simulink model "kde_old"  (R2022b)
settings: Solver=VariableStepAuto  StartTime=0.0  StopTime=orbit_E.T  FixedStep=1  RelTol=1e-9
values from neighbouring files (symbols this model uses):
  A0 = [1 0 0; 0 1 0; 0 0 1]    [test_script.m]
  gyro = struct('c', 15e-3, 'ARW', 0.15, 'sigma_b', deg2rad(0.3) / 3600,                'freq', 262, 'accuracy', 2.4e-9)    [test_script.m]
  H0 = sqrt((-29615e-9)^2+(-1728e-9)^2+(5186e-9)^2)    [test_script.m]
  I = [Ix; Iy; Iz]    [test_script.m]
  Ir = 0.005    [test_script.m]
  m_t = 5.9722e24    (= 5.9722e+24)    [test_script.m]
  Mr = 0    [test_script.m]
  orbit_E = struct('mu', astroConstants(13), 'a', astroConstants(23) + 2000,                    'e', 0.1, 'inc', deg2rad(10), 'G', astroConstants(1),                    'theta0', 0, 'R', astroConstants(23))    [test_script.m]
  orbit_S = struct('mu', astroConstants(4), 'a', astroConstants(2), 'e', 0.0167,                    'epsilon', deg2rad(23.45), 'G', astroConstants(1),                    'theta0', 0  )    [test_script.m]
  solarPanel = struct( 'r', r, 'P', radiation/(3e8),                      'rho_d', .1, 'rho_s', [.5, .5, .5, .5, .5 .5, .1, .1, .1, .1],                      'area', [.06 .06 .04 .06 .06 .04 .12 .12 .12 .12])    [test_script.m]
  w0 = [0; 0; orbit_E.n]    [test_script.m]
  wr0 = 0    [test_script.m]
undefined symbols (not defined in the file or in its folder): k1, k2
libraries: matrix_library x6, vrlib x2, dspinverses x1, simulink_extras x1
settings Model: Creator=stefa  LastModifiedBy=stefa
settings SolverCC: ZeroCrossAlgorithm=Adaptive

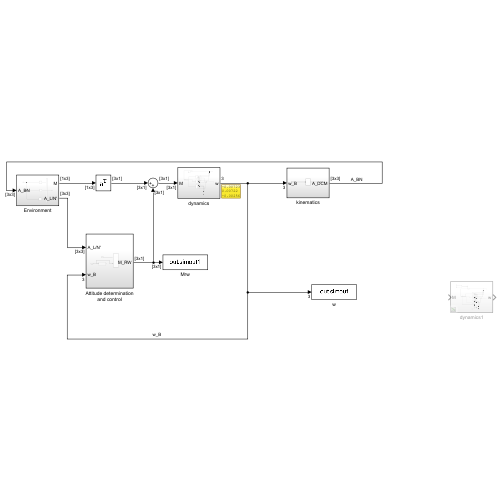
[thumbnail: Simulink's stored preview of the top-level diagram]
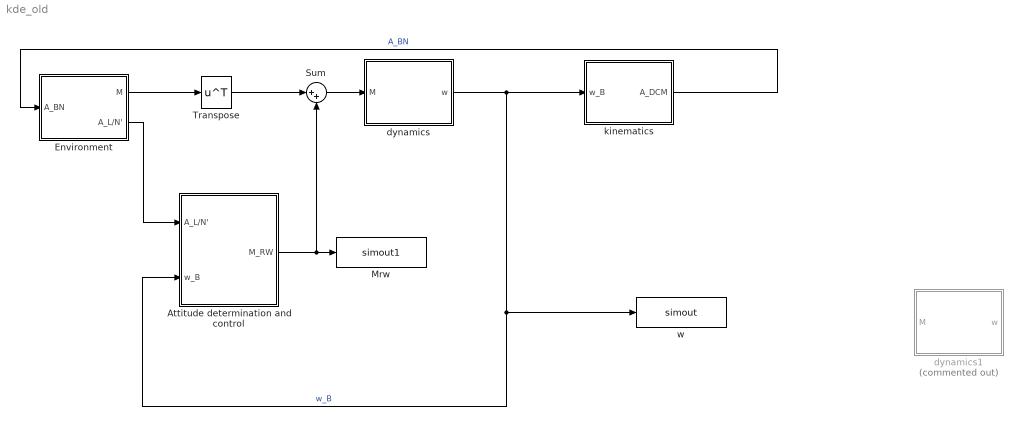
== system kde_old ==
  Attitude determination and control : Subsystem
  Environment : Subsystem
  Mrw : ToWorkspace  VariableName=simout1  SaveFormat=Timeseries  SampleTime=-1
  Sum : Sum  Inputs=|++
  Transpose : Math  Operator=transpose
  dynamics : Subsystem
  dynamics1 : Subsystem  Commented=on
  kinematics : Subsystem
  w : ToWorkspace  VariableName=simout  SaveFormat=Timeseries  SampleTime=-1
  wires:
  dynamics/1(w) -> kinematics/1(w_B), w/1, Attitude determination and control/2(w_B)  "w_B"
  kinematics/1(A_DCM) -> Environment/1(A_BN)  "A_BN"
  Sum/1 -> dynamics/1(M)
  Environment/2(A_L/N') -> Attitude determination and control/1(A_L/N')
  Attitude determination and control/1(M_RW) -> Mrw/1, Sum/2
  Environment/1(M) -> Transpose/1
  Transpose/1 -> Sum/1

== system kde_old/Attitude determination and control ==
  A_L/N' : Inport
  w_B : Inport  Port=2
  Actuator : Subsystem
  Sensors : Subsystem
  M_RW : Outport
  wires:
  A_L/N'/1 -> Actuator/1(A_L/N')
  Actuator/1(M_RW) -> M_RW/1
  w_B/1 -> Actuator/2(w_B), Sensors/1(w_B)
  Sensors/1(w_MB) -> Actuator/3(W_MB)

== system kde_old/Environment ==
  A_BN : Inport
  Magnetic field : Subsystem
  Sum : Sum  Inputs=+++
  gravity gradient : Subsystem
  srp disturbance : Subsystem
  M : Outport
  A_L/N' : Outport  Port=2
  wires:
  A_BN/1 -> Magnetic field/1(A_BN), srp disturbance/1(A_BN), gravity gradient/1(AB/N)
  Sum/1 -> M/1
  Magnetic field/1(M_B) -> Sum/1
  srp disturbance/1(M_srp) -> Sum/2
  gravity gradient/1(M_g) -> Sum/3
  gravity gradient/2(A_L/N') -> A_L/N'/1

== system kde_old/dynamics ==
  M : Inport
  Constant1 : Constant  Value=I
  Constant5 : Constant  Value=w0
  Demux : Demux  Outputs=3
  Demux1 : Demux  Outputs=3
  Demux2 : Demux  Outputs=3
  Integrator : Integrator  InitialConditionSource=external
  Mux : Mux  Inputs=3
  Subsystem : Subsystem
  Subsystem1 : Subsystem
  Subsystem2 : Subsystem
  w : Outport
  wires:
  Constant1/1 -> Demux1/1
  Demux1/2 -> Subsystem/4(Iy), Subsystem1/4(Iy), Subsystem2/4(Iy)  "Iy"
  Integrator/1 -> w/1, Demux/1  "w"
  Demux1/1 -> Subsystem/3(Ix), Subsystem1/3(Ix), Subsystem2/3(Ix)  "Ix"
  Demux2/2 -> Subsystem1/6(My)  "My"
  Demux1/3 -> Subsystem/5(Iz), Subsystem1/5(Iz), Subsystem2/5(Iz)  "Iz"
  Subsystem1/1(wy_dot) -> Mux/2
  Demux/1 -> Subsystem1/1(wx), Subsystem2/1(wx)  "wx"
  Subsystem2/1(wz_dot) -> Mux/3
  Demux2/3 -> Subsystem2/6(Mz)  "Mz"
  M/1 -> Demux2/1
  Demux/3 -> Subsystem1/2(wz), Subsystem/2(wz)  "wz"
  Demux/2 -> Subsystem2/2(wy), Subsystem/1(wy)  "wy"
  Demux2/1 -> Subsystem/6(Mx)  "Mx"
  Mux/1 -> Integrator/1  "w_dot"
  Subsystem/1(wx_dot) -> Mux/1
  Constant5/1 -> Integrator/2

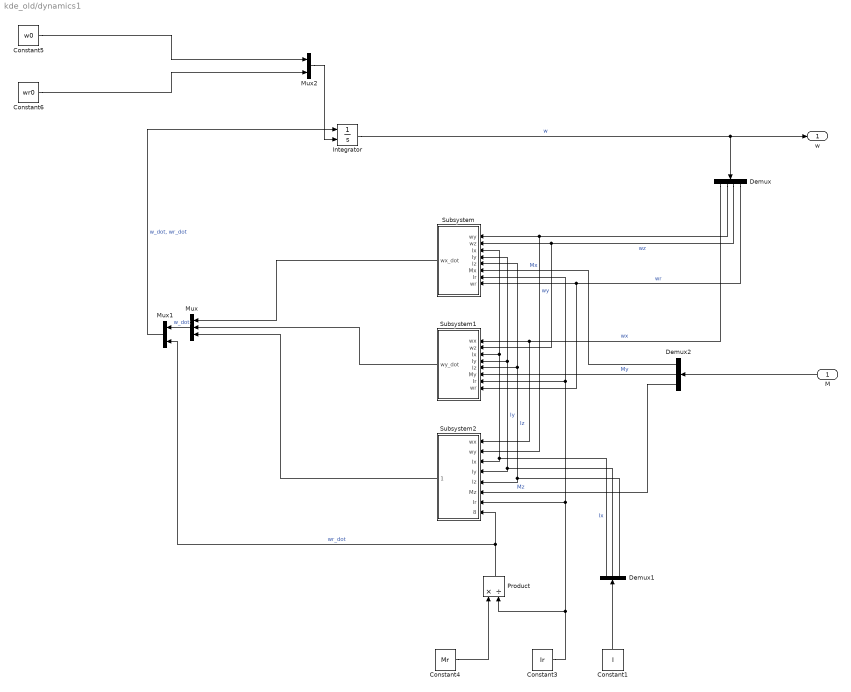
== system kde_old/dynamics1 ==
  M : Inport
  Constant1 : Constant  Value=I
  Constant3 : Constant  Value=Ir
  Constant4 : Constant  Value=Mr
  Constant5 : Constant  Value=w0
  Constant6 : Constant  Value=wr0
  Demux : Demux
  Demux1 : Demux  Outputs=3
  Demux2 : Demux  Outputs=3
  Integrator : Integrator  InitialConditionSource=external
  Mux : Mux  Inputs=3
  Mux1 : Mux  Inputs=2
  Mux2 : Mux  Inputs=2
  Product : Product  Inputs=*/
  Subsystem : Subsystem
  Subsystem1 : Subsystem
  Subsystem2 : Subsystem
  w : Outport
  wires:
  Constant1/1 -> Demux1/1
  Demux1/2 -> Subsystem/4(Iy), Subsystem1/4(Iy), Subsystem2/4(Iy)  "Iy"
  Integrator/1 -> w/1, Demux/1  "w"
  Demux1/1 -> Subsystem/3(Ix), Subsystem1/3(Ix), Subsystem2/3(Ix)  "Ix"
  Demux2/2 -> Subsystem1/6(My)  "My"
  Demux1/3 -> Subsystem/5(Iz), Subsystem1/5(Iz), Subsystem2/5(Iz)  "Iz"
  Subsystem1/1(wy_dot) -> Mux/2
  Demux/1 -> Subsystem1/1(wx), Subsystem2/1(wx)  "wx"
  Demux/4 -> Subsystem/8(wr), Subsystem1/8(wr)  "wr"
  Subsystem2/1(wz_dot) -> Mux/3
  Mux2/1 -> Integrator/2
  Demux2/3 -> Subsystem2/6(Mz)  "Mz"
  Constant6/1 -> Mux2/2
  M/1 -> Demux2/1
  Demux/3 -> Subsystem1/2(wz), Subsystem/2(wz)  "wz"
  Demux/2 -> Subsystem2/2(wy), Subsystem/1(wy)  "wy"
  Constant3/1 -> Product/2, Subsystem1/7(Ir), Subsystem/7(Ir), Subsystem2/7(Ir)
  Demux2/1 -> Subsystem/6(Mx)  "Mx"
  Mux1/1 -> Integrator/1  "w_dot, wr_dot"
  Product/1 -> Mux1/2, Subsystem2/8(wr_dot)  "wr_dot"
  Subsystem/1(wx_dot) -> Mux/1
  Constant5/1 -> Mux2/1
  Mux/1 -> Mux1/1  "w_dot"
  Constant4/1 -> Product/1

== system kde_old/kinematics ==
  w_B : Inport
  DCM : Subsystem
  A_DCM : Outport
  wires:
  w_B/1 -> DCM/1(w)
  DCM/1(A) -> A_DCM/1

== system kde_old/Attitude determination and control/Actuator ==
  A_L/N' : Inport
  w_B : Inport  Port=2
  W_MB : Inport  Port=3
  Constant : Constant  Value=[0 0 0]
  IdentityMatrix : IdentityMatrix  OutputDimensions=3
  IdentityMatrix1 : IdentityMatrix  OutputDimensions=3
  Reaction wheels : Subsystem
  Subsystem1 : Subsystem
  M_RW : Outport
  wires:
  IdentityMatrix/1 -> Reaction wheels/3(A)
  Reaction wheels/1(M_RW) -> M_RW/1
  Subsystem1/1(Mc) -> Reaction wheels/1(M_PD)
  Subsystem1/2(om) -> Reaction wheels/2(om)
  w_B/1 -> Subsystem1/2(w_MB)
  Constant/1 -> Subsystem1/3(w_target)
  IdentityMatrix1/1 -> Subsystem1/1(A_target)

== system kde_old/Attitude determination and control/Sensors ==
  w_B : Inport
  Constant : Constant  Commented=on  Value=gyro.c
  Constant1 : Constant  Commented=on  Value=gyro.A_eps
  MatrixMultiply1 : Product  Commented=on  Multiplication=Matrix(*)
  Product : Product  Commented=on
  noise : Subsystem
  w_MB : Outport
  wires:
  Product/1 -> MatrixMultiply1/1
  Constant1/1 -> Product/2
  Constant/1 -> Product/1
  noise/1(w_M) -> w_MB/1
  w_B/1 -> noise/1(C*A*w_B), MatrixMultiply1/2

== system kde_old/Environment/Magnetic field ==
  A_BN : Inport
  Cross Product : matrix_library/Cross Product
  Magnetic field : Subsystem
  m : Constant  Value=[0.01; 0.05; 0.01]
  M_B : Outport
  wires:
  A_BN/1 -> Magnetic field/1(A_BN)
  Magnetic field/1(b_B) -> Cross Product/2
  m/1 -> Cross Product/1
  Cross Product/1 -> M_B/1  "M_B"

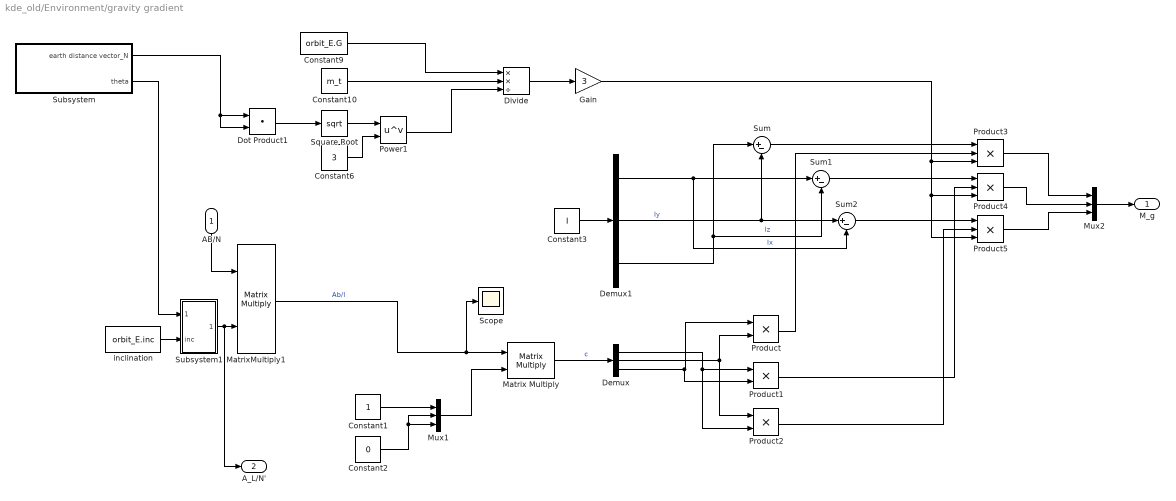
== system kde_old/Environment/gravity gradient ==
  AB/N : Inport
  Constant1 : Constant
  Constant10 : Constant  Value=m_t
  Constant2 : Constant  Value=0
  Constant3 : Constant  Value=I
  Constant6 : Constant  Value=3
  Constant9 : Constant  Value=orbit_E.G
  Demux : Demux  Outputs=3
  Demux1 : Demux  Outputs=3
  Divide : Product  Inputs=**/
  Dot Product1 : DotProduct  OutDataTypeStr=Inherit: Inherit via internal rule
  Gain : Gain  Gain=3
  Matrix Multiply : Product  Multiplication=Matrix(*)
  MatrixMultiply1 : Product  Multiplication=Matrix(*)
  Mux1 : Mux  Inputs=3
  Mux2 : Mux  Inputs=3
  Power1 : Math  Operator=pow
  Product : Product
  Product1 : Product
  Product2 : Product
  Product3 : Product  Inputs=3
  Product4 : Product  Inputs=3
  Product5 : Product  Inputs=3
  Scope : Scope
  Square Root : Sqrt
  Subsystem : Subsystem
  Subsystem1 : Subsystem
  Sum : Sum  Inputs=|+-
  Sum1 : Sum  Inputs=|+-
  Sum2 : Sum  Inputs=|+-
  inclination : Constant  Value=orbit_E.inc
  M_g : Outport
  A_L/N' : Outport  Port=2
  wires:
  AB/N/1 -> MatrixMultiply1/1
  MatrixMultiply1/1 -> Scope/1, Matrix Multiply/1  "Ab/l"
  Subsystem1/1(Al/n ') -> A_L/N'/1, MatrixMultiply1/2
  Subsystem/2(theta) -> Subsystem1/1(theta)
  Product4/1 -> Mux2/2
  Gain/1 -> Product5/3, Product4/3, Product3/3
  Demux1/2 -> Sum/2, Sum2/1  "Iy"
  Demux/3 -> Product1/2, Product/1
  Divide/1 -> Gain/1
  Demux1/3 -> Sum/1, Sum1/2  "Iz"
  Product1/1 -> Product4/2
  Constant1/1 -> Mux1/1
  Sum2/1 -> Product5/1
  Square Root/1 -> Power1/1
  Matrix Multiply/1 -> Demux/1  "c"
  Constant9/1 -> Divide/1
  Sum/1 -> Product3/1
  Demux/2 -> Product/2, Product2/1
  Constant6/1 -> Power1/2
  Product3/1 -> Mux2/1
  Mux1/1 -> Matrix Multiply/2
  Product/1 -> Product3/2
  Constant10/1 -> Divide/2
  Demux1/1 -> Sum2/2, Sum1/1  "Ix"
  Product2/1 -> Product5/2
  Constant2/1 -> Mux1/3, Mux1/2
  Product5/1 -> Mux2/3
  Demux/1 -> Product2/2, Product1/1
  Sum1/1 -> Product4/1
  Power1/1 -> Divide/3
  Dot Product1/1 -> Square Root/1
  Mux2/1 -> M_g/1
  Subsystem/1(earth distance vector_N) -> Dot Product1/2, Dot Product1/1
  Constant3/1 -> Demux1/1
  inclination/1 -> Subsystem1/2(inc)

== system kde_old/Environment/srp disturbance ==
  A_BN : Inport
  MatrixMultiply : Product  Multiplication=Matrix(*)
  Normalize Vector : vrlib/Utilities/Normalize Vector  maxzero=0
  Subsystem : Subsystem
  orientation s/c and solar panels : Subsystem
  sun distance magnitude : Subsystem
  M_srp : Outport
  wires:
  sun distance magnitude/1(S_N) -> Normalize Vector/1
  A_BN/1 -> MatrixMultiply/1
  Normalize Vector/1 -> MatrixMultiply/2
  Subsystem/1(M_SRP) -> M_srp/1
  orientation s/c and solar panels/1(N_B) -> Subsystem/2(N_B)
  MatrixMultiply/1 -> Subsystem/1(S_B)  "S_B"

== system kde_old/dynamics/Subsystem ==
  wy : Inport
  wz : Inport  Port=2
  Ix : Inport  Port=3
  Iy : Inport  Port=4
  Iz : Inport  Port=5
  Mx : Inport  Port=6
  Product : Product
  Product1 : Product
  Product3 : Product  Inputs=*/
  Sum : Sum  Inputs=|+-
  Sum1 : Sum  Inputs=|++
  wx_dot : Outport
  wires:
  Product1/1 -> Sum1/1
  Product/1 -> Product1/1
  Sum/1 -> Product1/2
  Product3/1 -> wx_dot/1  "wx_dot"
  Iy/1 -> Sum/1
  Iz/1 -> Sum/2
  wz/1 -> Product/1
  wy/1 -> Product/2
  Sum1/1 -> Product3/1
  Ix/1 -> Product3/2
  Mx/1 -> Sum1/2

== system kde_old/dynamics/Subsystem1 ==
  wx : Inport
  wz : Inport  Port=2
  Ix : Inport  Port=3
  Iy : Inport  Port=4
  Iz : Inport  Port=5
  My : Inport  Port=6
  Product : Product
  Product1 : Product
  Product3 : Product  Inputs=*/
  Sum : Sum  Inputs=|+-
  Sum2 : Sum  Inputs=|++
  wy_dot : Outport
  wires:
  Sum2/1 -> Product3/1
  Product1/1 -> Sum2/1
  Iy/1 -> Product3/2
  Sum/1 -> Product1/2
  Iz/1 -> Sum/1
  Product/1 -> Product1/1
  Product3/1 -> wy_dot/1
  Ix/1 -> Sum/2
  My/1 -> Sum2/2
  wz/1 -> Product/1
  wx/1 -> Product/2

== system kde_old/dynamics/Subsystem2 ==
  wx : Inport
  wy : Inport  Port=2
  Ix : Inport  Port=3
  Iy : Inport  Port=4
  Iz : Inport  Port=5
  Mz : Inport  Port=6
  Product : Product
  Product1 : Product
  Product3 : Product  Inputs=*/
  Sum : Sum  Inputs=|+-
  Sum1 : Sum  Inputs=|++
  wz_dot : Outport
  wires:
  Sum/1 -> Product1/2
  Product/1 -> Product1/1
  Iz/1 -> Product3/2
  Product3/1 -> wz_dot/1  "wz_dot"
  Sum1/1 -> Product3/1
  Product1/1 -> Sum1/1
  Ix/1 -> Sum/1
  wy/1 -> Product/1
  Iy/1 -> Sum/2
  Mz/1 -> Sum1/2
  wx/1 -> Product/2

== system kde_old/dynamics1/Subsystem ==
  wy : Inport
  wz : Inport  Port=2
  Ix : Inport  Port=3
  Iy : Inport  Port=4
  Iz : Inport  Port=5
  Mx : Inport  Port=6
  Ir : Inport  Port=7
  wr : Inport  Port=8
  Product : Product
  Product1 : Product
  Product2 : Product  Inputs=3
  Product3 : Product  Inputs=*/
  Sum : Sum  Inputs=|+-
  Sum1 : Sum  Inputs=|+-+
  wx_dot : Outport
  wires:
  Product1/1 -> Sum1/1
  Product/1 -> Product1/1
  Product2/1 -> Sum1/2
  Ir/1 -> Product2/2
  Sum/1 -> Product1/2
  Product3/1 -> wx_dot/1  "wx_dot"
  Iy/1 -> Sum/1
  Iz/1 -> Sum/2
  wz/1 -> Product/1
  Mx/1 -> Sum1/3
  wy/1 -> Product2/1, Product/2
  Sum1/1 -> Product3/1
  Ix/1 -> Product3/2
  wr/1 -> Product2/3

== system kde_old/dynamics1/Subsystem1 ==
  wx : Inport
  wz : Inport  Port=2
  Ix : Inport  Port=3
  Iy : Inport  Port=4
  Iz : Inport  Port=5
  My : Inport  Port=6
  Ir : Inport  Port=7
  wr : Inport  Port=8
  Product : Product
  Product1 : Product
  Product2 : Product  Inputs=3
  Product3 : Product  Inputs=*/
  Sum : Sum  Inputs=|+-
  Sum1 : Sum  Inputs=|++
  Sum2 : Sum  Inputs=|++
  wy_dot : Outport
  wires:
  Product1/1 -> Sum1/1
  Product2/1 -> Sum1/2
  Sum2/1 -> Product3/1
  Sum1/1 -> Sum2/1
  Iy/1 -> Product3/2
  Sum/1 -> Product1/2
  Iz/1 -> Sum/1
  Product/1 -> Product1/1
  Product3/1 -> wy_dot/1
  Ix/1 -> Sum/2
  My/1 -> Sum2/2
  wz/1 -> Product/1
  wx/1 -> Product2/1, Product/2
  wr/1 -> Product2/2
  Ir/1 -> Product2/3

== system kde_old/dynamics1/Subsystem2 ==
  wx : Inport
  wy : Inport  Port=2
  Ix : Inport  Port=3
  Iy : Inport  Port=4
  Iz : Inport  Port=5
  Mz : Inport  Port=6
  Ir : Inport  Port=7
  wr_dot : Inport  Port=8
  Product : Product
  Product1 : Product
  Product2 : Product
  Product3 : Product  Inputs=*/
  Sum : Sum  Inputs=|+-
  Sum1 : Sum  Inputs=|+-+
  wz_dot : Outport
  wires:
  Sum/1 -> Product1/2
  Product/1 -> Product1/1
  Iz/1 -> Product3/2
  Product3/1 -> wz_dot/1  "wz_dot"
  Sum1/1 -> Product3/1
  Product2/1 -> Sum1/2
  Product1/1 -> Sum1/1
  Ix/1 -> Sum/1
  wy/1 -> Product/1
  Iy/1 -> Sum/2
  Mz/1 -> Sum1/3
  Ir/1 -> Product2/1
  wx/1 -> Product/2
  wr_dot/1 -> Product2/2

== system kde_old/kinematics/DCM ==
  w : Inport
  Constant : Constant  Value=0
  Constant1 : Constant  Value=A0
  Gain : Gain  Gain=3/2
  Gain1 : Gain  Gain=1/2
  Integrator : Integrator  InitialConditionSource=external
  MatrixMultiply : Product  Multiplication=Matrix(*)
  MatrixMultiply1 : Product  Inputs=3  Multiplication=Matrix(*)
  Subsystem : Subsystem
  Sum : Sum  Inputs=|-+
  Transpose : Math  Operator=transpose
  A : Outport
  wires:
  Sum/1 -> A/1, MatrixMultiply/2
  Transpose/1 -> MatrixMultiply1/2
  MatrixMultiply/1 -> Integrator/1  "A_dot"
  Integrator/1 -> MatrixMultiply1/3, Gain/1, Transpose/1, MatrixMultiply1/1  "A"
  Subsystem/1(-[om^]) -> MatrixMultiply/1
  MatrixMultiply1/1 -> Gain1/1
  Constant/1 -> Subsystem/2(0)
  w/1 -> Subsystem/1(w)
  Constant1/1 -> Integrator/2
  Gain1/1 -> Sum/1
  Gain/1 -> Sum/2

== system kde_old/Attitude determination and control/Actuator/Reaction wheels ==
  M_PD : Inport
  om : Inport  Port=2
  A : Inport  Port=3
  Cross Product : matrix_library/Cross Product
  RW dynamics : Subsystem
  Sum : Sum  Inputs=|--
  M_RW : Outport
  wires:
  M_PD/1 -> RW dynamics/1(M_PD)
  om/1 -> Cross Product/1, RW dynamics/2(om)
  A/1 -> RW dynamics/3(A)
  RW dynamics/1(hr_dot) -> Sum/1
  RW dynamics/2(hr) -> Cross Product/2
  Cross Product/1 -> Sum/2
  Sum/1 -> M_RW/1

== system kde_old/Attitude determination and control/Actuator/Subsystem1 ==
  A_target : Inport
  w_MB : Inport  Port=2
  w_target : Inport  Port=3
  Constant : Constant  Value=I
  Constant1 : Constant  Value=k1
  Constant2 : Constant  Value=k2
  IdentityMatrix : IdentityMatrix  OutputDimensions=3
  Integrator : Integrator
  Integrator1 : Integrator  InitialConditionSource=external
  MATLAB Function : MATLAB Function  TreatAsAtomicUnit=on
  MATLAB Function1 : MATLAB Function  TreatAsAtomicUnit=on
  MATLAB Function2 : MATLAB Function  TreatAsAtomicUnit=on
  MatrixMultiply : Product  Multiplication=Matrix(*)
  Sum : Sum  Inputs=-+|
  Mc : Outport
  om : Outport  Port=2
  wires:
  Integrator/1 -> om/1, MATLAB Function1/1(om), MATLAB Function/3(om)
  MATLAB Function/1(om_dot) -> Integrator/1
  Constant/1 -> MATLAB Function/1(I)
  MATLAB Function1/1(dA) -> Integrator1/1
  Integrator1/1 -> MATLAB Function1/2(A), MatrixMultiply/1
  IdentityMatrix/1 -> Integrator1/2
  A_target/1 -> MatrixMultiply/2
  MatrixMultiply/1 -> MATLAB Function2/2(Ae)  "Ae"
  MATLAB Function2/1(u) -> MATLAB Function/2(u), Mc/1
  Constant1/1 -> MATLAB Function2/3(k1)
  Constant2/1 -> MATLAB Function2/4(k2)
  w_target/1 -> Sum/1
  w_MB/1 -> Sum/2
  Sum/1 -> MATLAB Function2/1(om)

== system kde_old/Attitude determination and control/Sensors/noise ==
  C*A*w_B : Inport
  Integrator : Integrator
  Sum : Sum  Inputs=+++
  b_dot : RandomNumber  Variance=(gyro.sigma_b) ^2  SampleTime=2000
  n : RandomNumber  Variance=(deg2rad(gyro.ARW)/60 * sqrt(gyro.freq))^2  SampleTime=2000
  w_M : Outport
  wires:
  b_dot/1 -> Integrator/1
  Sum/1 -> w_M/1
  n/1 -> Sum/2
  Integrator/1 -> Sum/3  "b"
  C*A*w_B/1 -> Sum/1

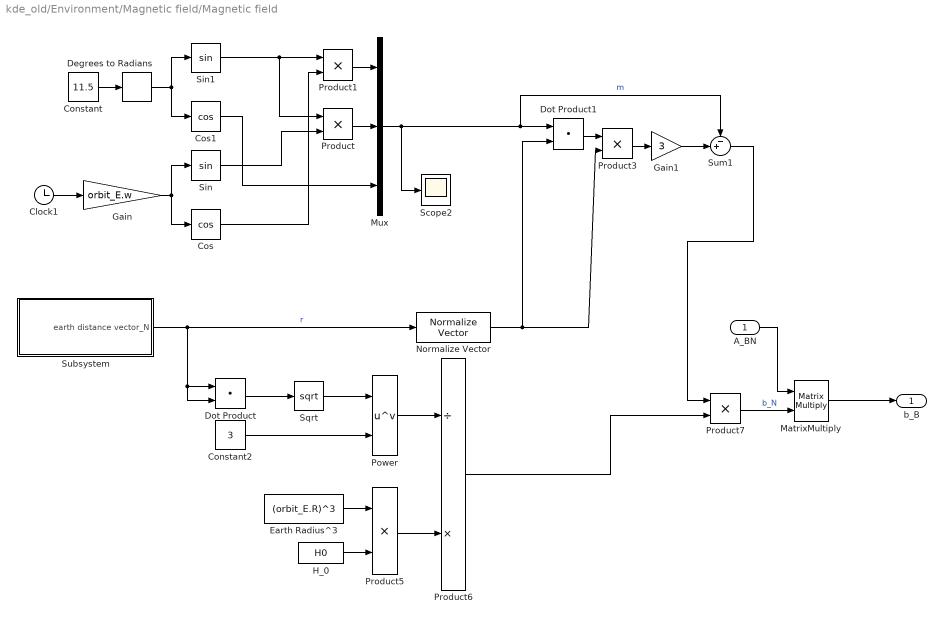
== system kde_old/Environment/Magnetic field/Magnetic field ==
  A_BN : Inport
  Clock1 : Clock
  Constant : Constant  Value=11.5
  Constant2 : Constant  Value=3
  Cos : Trigonometry  Operator=cos
  Cos1 : Trigonometry  Operator=cos
  Degrees to Radians : simulink_extras/Transformations/Degrees to Radians
  Dot Product : DotProduct  OutDataTypeStr=Inherit: Inherit via internal rule
  Dot Product1 : DotProduct  OutDataTypeStr=Inherit: Inherit via internal rule
  Earth Radius^3 : Constant  Value=(orbit_E.R)^3
  Gain : Gain  Gain=orbit_E.w
  Gain1 : Gain  Gain=3
  H_0 : Constant  Value=H0
  MatrixMultiply : Product  Multiplication=Matrix(*)
  Mux : Mux  Inputs=3
  Normalize Vector : vrlib/Utilities/Normalize Vector  maxzero=0
  Power : Math  Operator=pow
  Product{,1,3,5,7} (5 alike) : Product
  Product6 : Product  Inputs=/*
  Scope2 : Scope
  Sin : Trigonometry
  Sin1 : Trigonometry
  Sqrt : Sqrt
  Subsystem : Subsystem
  Sum1 : Sum  Inputs=-+|
  b_B : Outport
  wires:
  Constant2/1 -> Power/2
  Clock1/1 -> Gain/1
  Product1/1 -> Mux/1
  H_0/1 -> Product5/2
  Gain/1 -> Cos/1, Sin/1
  Subsystem/1(earth distance vector_N) -> Normalize Vector/1, Dot Product/1, Dot Product/2  "r"
  Mux/1 -> Dot Product1/1, Sum1/1, Scope2/1  "m"
  Dot Product/1 -> Sqrt/1
  Power/1 -> Product6/1
  Normalize Vector/1 -> Dot Product1/2, Product3/2
  Product6/1 -> Product7/2
  Dot Product1/1 -> Product3/1
  Product3/1 -> Gain1/1
  Degrees to Radians/1 -> Cos1/1, Sin1/1
  Cos1/1 -> Mux/3
  Product5/1 -> Product6/2
  Earth Radius^3/1 -> Product5/1
  Product/1 -> Mux/2
  Constant/1 -> Degrees to Radians/1
  Sin1/1 -> Product/1, Product1/1
  Sin/1 -> Product/2
  Product7/1 -> MatrixMultiply/2  "b_N"
  A_BN/1 -> MatrixMultiply/1
  MatrixMultiply/1 -> b_B/1
  Sqrt/1 -> Power/1
  Cos/1 -> Product1/2
  Sum1/1 -> Product7/1
  Gain1/1 -> Sum1/2

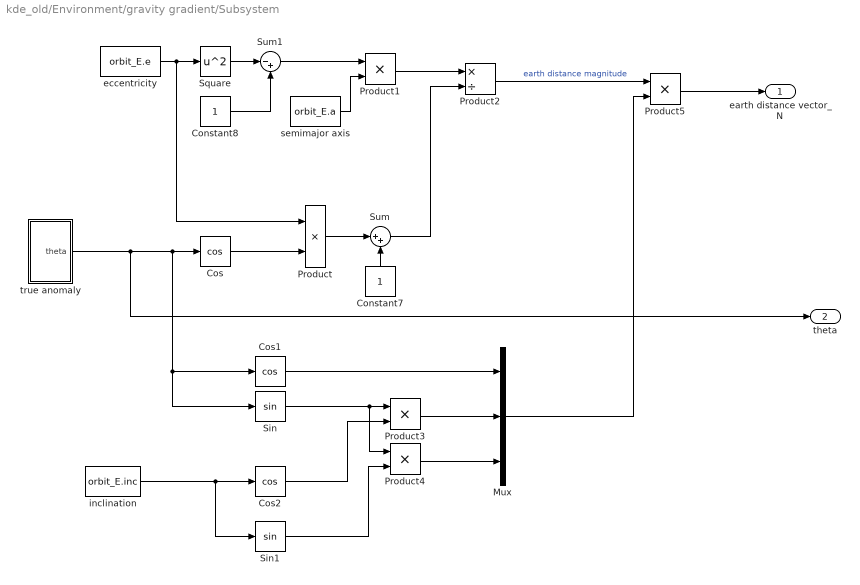
== system kde_old/Environment/gravity gradient/Subsystem ==
  Constant7 : Constant
  Constant8 : Constant
  Cos : Trigonometry  Operator=cos
  Cos1 : Trigonometry  Operator=cos
  Cos2 : Trigonometry  Operator=cos
  Mux : Mux  Inputs=3
  Product{,1,3..5} (5 alike) : Product
  Product2 : Product  Inputs=*/
  Sin : Trigonometry
  Sin1 : Trigonometry
  Square : Math  Operator=square
  Sum : Sum  Inputs=|++
  Sum1 : Sum  Inputs=|-+
  eccentricity : Constant  Value=orbit_E.e
  inclination : Constant  Value=orbit_E.inc
  semimajor axis : Constant  Value=orbit_E.a
  true anomaly : Subsystem
  earth distance vector_N : Outport
  theta : Outport  Port=2
  wires:
  Mux/1 -> Product5/2
  Product2/1 -> Product5/1  "earth distance magnitude"
  Product1/1 -> Product2/1
  Constant8/1 -> Sum1/2
  Sin/1 -> Product3/1, Product4/1
  true anomaly/1(theta) -> theta/1, Sin/1, Cos1/1, Cos/1
  Cos/1 -> Product/2
  eccentricity/1 -> Product/1, Square/1
  Sin1/1 -> Product4/2
  Sum1/1 -> Product1/1
  Sum/1 -> Product2/2
  Product3/1 -> Mux/2
  Cos1/1 -> Mux/1
  Square/1 -> Sum1/1
  semimajor axis/1 -> Product1/2
  inclination/1 -> Sin1/1, Cos2/1
  Product4/1 -> Mux/3
  Constant7/1 -> Sum/2
  Product/1 -> Sum/1
  Product5/1 -> earth distance vector_N/1
  Cos2/1 -> Product3/2

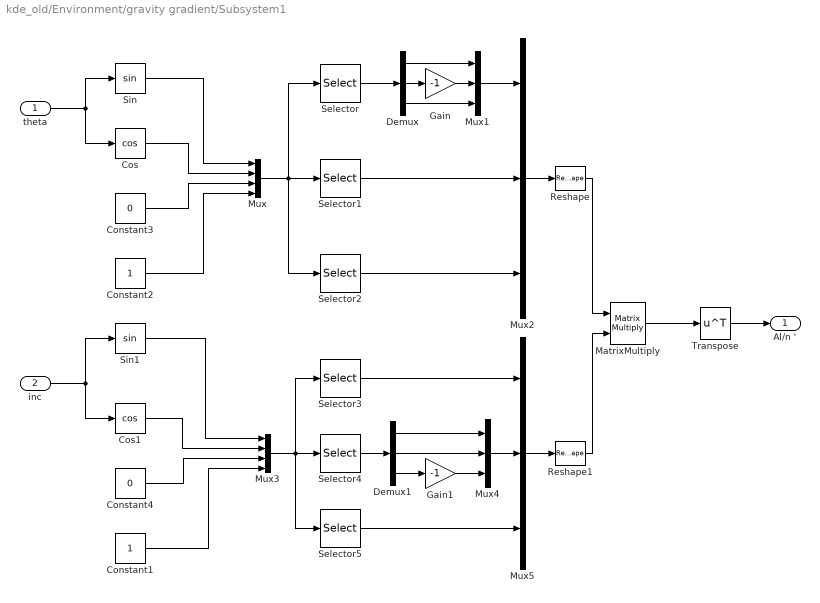
== system kde_old/Environment/gravity gradient/Subsystem1 ==
  theta : Inport
  inc : Inport  Port=2
  Constant1 : Constant
  Constant2 : Constant
  Constant3 : Constant  Value=0
  Constant4 : Constant  Value=0
  Cos : Trigonometry  Operator=cos
  Cos1 : Trigonometry  Operator=cos
  Demux : Demux  Outputs=3
  Demux1 : Demux  Outputs=3
  Gain : Gain  Gain=-1
  Gain1 : Gain  Gain=-1
  MatrixMultiply : Product  Multiplication=Matrix(*)
  Mux : Mux
  Mux{1..2,4..5} (4 alike) : Mux  Inputs=3
  Mux3 : Mux
  Reshape : Reshape  OutputDimensionality=Customize  OutputDimensions=[3,3]
  Reshape1 : Reshape  OutputDimensionality=Customize  OutputDimensions=[3,3]
  Selector : Selector  InputPortWidth=4  IndexOptions=Index vector (dialog)  Indices=[2 1 3]  OutputSizes=1
  Selector1 : Selector  InputPortWidth=4  IndexOptions=Index vector (dialog)  Indices=[1 2 3]  OutputSizes=1
  Selector2 : Selector  InputPortWidth=4  IndexOptions=Index vector (dialog)  Indices=[3 3 4]  OutputSizes=1
  Selector3 : Selector  InputPortWidth=4  IndexOptions=Index vector (dialog)  Indices=[4 3 3]  OutputSizes=1
  Selector4 : Selector  InputPortWidth=4  IndexOptions=Index vector (dialog)  Indices=[3 2 1]  OutputSizes=1
  Selector5 : Selector  InputPortWidth=4  IndexOptions=Index vector (dialog)  Indices=[3 1 2]  OutputSizes=1
  Sin : Trigonometry
  Sin1 : Trigonometry
  Transpose : Math  Operator=transpose
  Al/n ' : Outport
  wires:
  Constant2/1 -> Mux/4
  Constant3/1 -> Mux/3
  theta/1 -> Cos/1, Sin/1
  Cos/1 -> Mux/2
  Sin/1 -> Mux/1
  Mux/1 -> Selector2/1, Selector1/1, Selector/1
  Selector/1 -> Demux/1
  Demux/2 -> Gain/1
  Gain/1 -> Mux1/2
  Demux/3 -> Mux1/3
  Demux/1 -> Mux1/1
  Selector2/1 -> Mux2/3
  Mux1/1 -> Mux2/1
  Selector1/1 -> Mux2/2
  Mux2/1 -> Reshape/1
  Cos1/1 -> Mux3/2
  Sin1/1 -> Mux3/1
  Constant4/1 -> Mux3/3
  Constant1/1 -> Mux3/4
  inc/1 -> Cos1/1, Sin1/1
  Selector4/1 -> Demux1/1
  Demux1/3 -> Gain1/1
  Demux1/2 -> Mux4/2
  Demux1/1 -> Mux4/1
  Gain1/1 -> Mux4/3
  Mux3/1 -> Selector3/1, Selector4/1, Selector5/1
  Mux4/1 -> Mux5/2
  Selector3/1 -> Mux5/1
  Selector5/1 -> Mux5/3
  Mux5/1 -> Reshape1/1
  Reshape/1 -> MatrixMultiply/1
  Reshape1/1 -> MatrixMultiply/2
  MatrixMultiply/1 -> Transpose/1
  Transpose/1 -> Al/n '/1

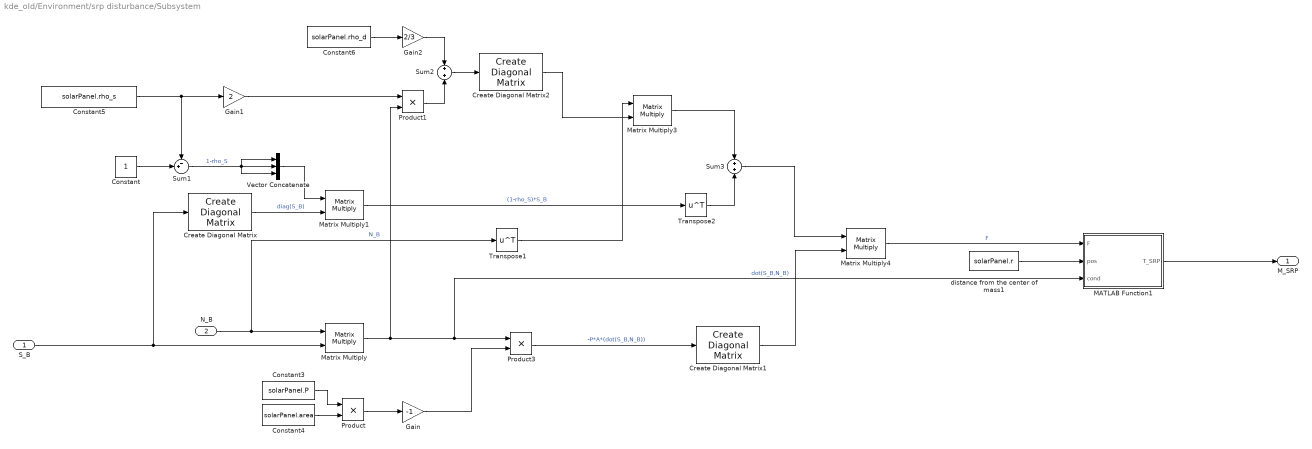
== system kde_old/Environment/srp disturbance/Subsystem ==
  S_B : Inport
  N_B : Inport  Port=2
  Constant : Constant
  Constant3 : Constant  Value=solarPanel.P
  Constant4 : Constant  Value=solarPanel.area
  Constant5 : Constant  Value=solarPanel.rho_s
  Constant6 : Constant  Value=solarPanel.rho_d
  Create Diagonal Matrix : matrix_library/Create Diagonal Matrix
      settings: LibrarySourceBlock=|
      | simulink/Matrix
      | Operations/Create Diagonal
      | Matrix
  Create Diagonal Matrix1 : matrix_library/Create Diagonal Matrix
      settings: LibrarySourceBlock=|
      | simulink/Matrix
      | Operations/Create Diagonal
      | Matrix
  Create Diagonal Matrix2 : matrix_library/Create Diagonal Matrix
      settings: LibrarySourceBlock=|
      | simulink/Matrix
      | Operations/Create Diagonal
      | Matrix
  Gain : Gain  Gain=-1
  Gain1 : Gain  Gain=2
  Gain2 : Gain  Gain=2/3
  MATLAB Function1 : MATLAB Function  TreatAsAtomicUnit=on
  Matrix Multiply{,1,3..4} (4 alike) : Product  Multiplication=Matrix(*)
  Product : Product
  Product1 : Product
  Product3 : Product
  Sum1 : Sum  Inputs=-+|
  Sum2 : Sum
  Sum3 : Sum
  Transpose1 : Math  Operator=transpose
  Transpose2 : Math  Operator=transpose
  Vector Concatenate : Concatenate  NumInputs=3  Mode=Multidimensional array  ConcatenateDimension=2
  distance from the center of mass1 : Constant  Value=solarPanel.r
  M_SRP : Outport
  wires:
  MATLAB Function1/1(T_SRP) -> M_SRP/1
  Create Diagonal Matrix1/1 -> Matrix Multiply4/2
  Product/1 -> Gain/1
  Matrix Multiply3/1 -> Sum3/1
  Product1/1 -> Sum2/2
  Transpose2/1 -> Sum3/2
  S_B/1 -> Create Diagonal Matrix/1, Matrix Multiply/2
  Constant4/1 -> Product/2
  Create Diagonal Matrix2/1 -> Matrix Multiply3/2
  Gain2/1 -> Sum2/1
  Constant/1 -> Sum1/2
  Matrix Multiply4/1 -> MATLAB Function1/1(F)  "F"
  Sum2/1 -> Create Diagonal Matrix2/1
  Product3/1 -> Create Diagonal Matrix1/1  "-P*A*(dot(S_B,N_B))"
  Create Diagonal Matrix/1 -> Matrix Multiply1/2  "diag(S_B)"
  N_B/1 -> Transpose1/1, Matrix Multiply/1  "N_B"
  Constant3/1 -> Product/1
  distance from the center of mass1/1 -> MATLAB Function1/2(pos)
  Matrix Multiply1/1 -> Transpose2/1  "(1-rho_S)*S_B"
  Constant5/1 -> Gain1/1, Sum1/1
  Gain/1 -> Product3/2
  Constant6/1 -> Gain2/1
  Sum1/1 -> Vector Concatenate/1, Vector Concatenate/3, Vector Concatenate/2  "1-rho_S"
  Gain1/1 -> Product1/1
  Sum3/1 -> Matrix Multiply4/1
  Matrix Multiply/1 -> Product1/2, MATLAB Function1/3(cond), Product3/1  "dot(S_B,N_B)"
  Vector Concatenate/1 -> Matrix Multiply1/1
  Transpose1/1 -> Matrix Multiply3/1

== system kde_old/Environment/srp disturbance/orientation s//c and solar panels ==
  Transpose : Math  Operator=transpose
  Vector Concatenate : Concatenate  NumInputs=10  Mode=Multidimensional array  ConcatenateDimension=2
  orientation s/c and solar panels in B : Subsystem
  N_B : Outport
  wires:
  orientation s/c and solar panels in B/6(n6) -> Vector Concatenate/6
  orientation s/c and solar panels in B/7(n7) -> Vector Concatenate/7
  orientation s/c and solar panels in B/3(n3) -> Vector Concatenate/3
  orientation s/c and solar panels in B/5(n5) -> Vector Concatenate/5
  orientation s/c and solar panels in B/10(n10) -> Vector Concatenate/10
  orientation s/c and solar panels in B/2(n2) -> Vector Concatenate/2
  orientation s/c and solar panels in B/8(n8) -> Vector Concatenate/8
  orientation s/c and solar panels in B/1(n1) -> Vector Concatenate/1
  orientation s/c and solar panels in B/4(n4) -> Vector Concatenate/4
  orientation s/c and solar panels in B/9(n9) -> Vector Concatenate/9
  Vector Concatenate/1 -> Transpose/1  "N_B"
  Transpose/1 -> N_B/1

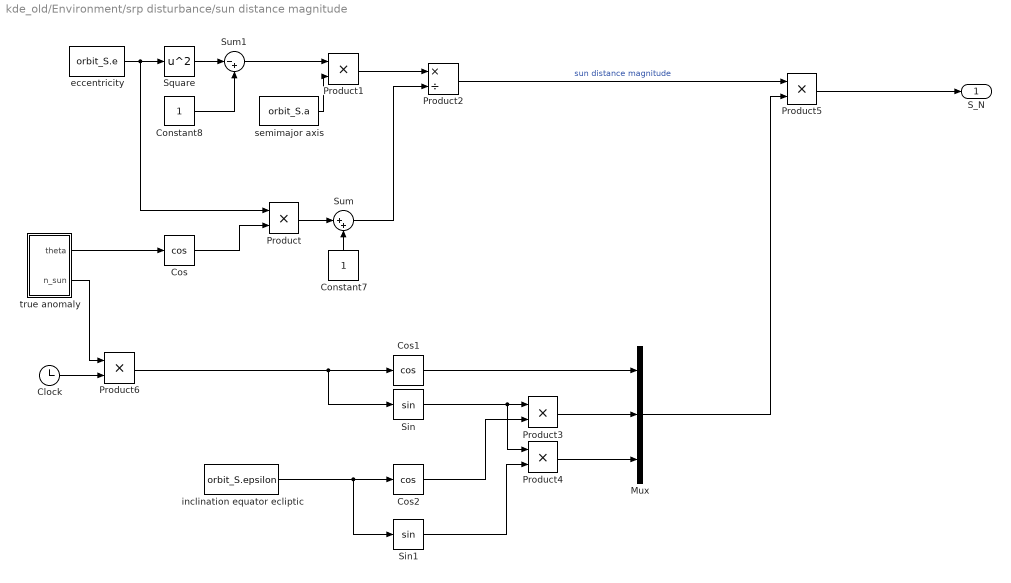
== system kde_old/Environment/srp disturbance/sun distance magnitude ==
  Clock : Clock
  Constant7 : Constant
  Constant8 : Constant
  Cos : Trigonometry  Operator=cos
  Cos1 : Trigonometry  Operator=cos
  Cos2 : Trigonometry  Operator=cos
  Mux : Mux  Inputs=3
  Product{,1,3..6} (6 alike) : Product
  Product2 : Product  Inputs=*/
  Sin : Trigonometry
  Sin1 : Trigonometry
  Square : Math  Operator=square
  Sum : Sum  Inputs=|++
  Sum1 : Sum  Inputs=|-+
  eccentricity : Constant  Value=orbit_S.e
  inclination equator ecliptic : Constant  Value=orbit_S.epsilon
  semimajor axis : Constant  Value=orbit_S.a
  true anomaly : Subsystem
  S_N : Outport
  wires:
  Mux/1 -> Product5/2
  Product2/1 -> Product5/1  "sun distance magnitude"
  Product1/1 -> Product2/1
  Constant8/1 -> Sum1/2
  Sin/1 -> Product4/1, Product3/1
  Cos/1 -> Product/2
  eccentricity/1 -> Product/1, Square/1
  Sin1/1 -> Product4/2
  Sum1/1 -> Product1/1
  Product3/1 -> Mux/2
  Cos1/1 -> Mux/1
  Square/1 -> Sum1/1
  semimajor axis/1 -> Product1/2
  inclination equator ecliptic/1 -> Sin1/1, Cos2/1
  Product4/1 -> Mux/3
  Constant7/1 -> Sum/2
  Product/1 -> Sum/1
  Cos2/1 -> Product3/2
  true anomaly/1(theta) -> Cos/1
  Clock/1 -> Product6/2
  true anomaly/2(n_sun) -> Product6/1
  Product6/1 -> Sin/1, Cos1/1
  Sum/1 -> Product2/2
  Product5/1 -> S_N/1

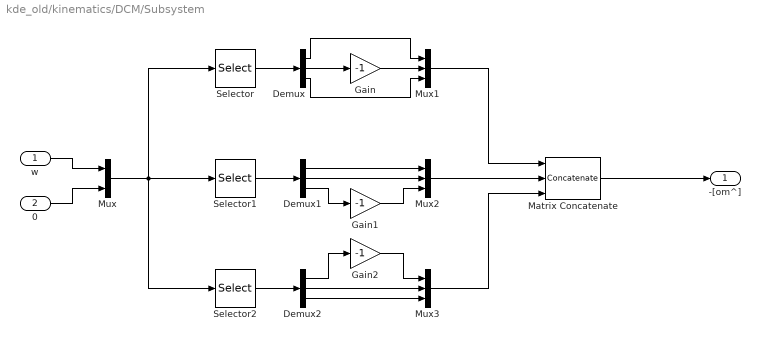
== system kde_old/kinematics/DCM/Subsystem ==
  w : Inport
  0 : Inport  Port=2
  Demux : Demux  Outputs=3
  Demux1 : Demux  Outputs=3
  Demux2 : Demux  Outputs=3
  Gain : Gain  Gain=-1
  Gain1 : Gain  Gain=-1
  Gain2 : Gain  Gain=-1
  Matrix Concatenate : Concatenate  NumInputs=3  Mode=Multidimensional array  ConcatenateDimension=2
  Mux : Mux  Inputs=2
  Mux1 : Mux  Inputs=3
  Mux2 : Mux  Inputs=3
  Mux3 : Mux  Inputs=3
  Selector : Selector  InputPortWidth=4  IndexOptions=Index vector (dialog)  Indices=[4 3 2]  OutputSizes=1
  Selector1 : Selector  InputPortWidth=4  IndexOptions=Index vector (dialog)  Indices=[3 4 1]  OutputSizes=1
  Selector2 : Selector  InputPortWidth=4  IndexOptions=Index vector (dialog)  Indices=[2 1 4]  OutputSizes=1
  -[om^] : Outport
  wires:
  w/1 -> Mux/1
  Demux/3 -> Mux1/3
  Demux/1 -> Mux1/1
  Demux2/3 -> Mux3/3
  Selector2/1 -> Demux2/1
  Mux/1 -> Selector2/1, Selector1/1, Selector/1
  Selector/1 -> Demux/1
  Demux/2 -> Gain/1
  Mux3/1 -> Matrix Concatenate/3
  Mux1/1 -> Matrix Concatenate/1
  Demux2/2 -> Mux3/2
  Gain1/1 -> Mux2/3
  Selector1/1 -> Demux1/1
  Demux1/2 -> Mux2/2
  Demux1/3 -> Gain1/1
  Gain/1 -> Mux1/2
  Mux2/1 -> Matrix Concatenate/2
  Demux1/1 -> Mux2/1
  Demux2/1 -> Gain2/1
  Gain2/1 -> Mux3/1
  Matrix Concatenate/1 -> -[om^]/1
  0/1 -> Mux/2

== system kde_old/Attitude determination and control/Actuator/Reaction wheels/RW dynamics ==
  M_PD : Inport
  om : Inport  Port=2
  A : Inport  Port=3
  Cross Product : matrix_library/Cross Product
  Gain : Gain  Gain=-1
  Integrator : Integrator
  MatrixMultiply : Product  Multiplication=Matrix(*)
  MatrixMultiply1 : Product  Multiplication=Matrix(*)
  Pseudoinverse : dspinverses/Pseudoinverse  wanterr=off  SimulateUsing=Interpreted execution
  Sum : Sum  Inputs=|++
  hr_dot : Outport
  hr : Outport  Port=2
  wires:
  A/1 -> MatrixMultiply/1, Pseudoinverse/1
  Integrator/1 -> hr/1, MatrixMultiply/2  "hr"
  Gain/1 -> hr_dot/1, Integrator/1  "hr_dot"
  M_PD/1 -> Sum/2
  Pseudoinverse/1 -> MatrixMultiply1/1
  Sum/1 -> MatrixMultiply1/2
  MatrixMultiply1/1 -> Gain/1
  MatrixMultiply/1 -> Cross Product/2
  Cross Product/1 -> Sum/1
  om/1 -> Cross Product/1

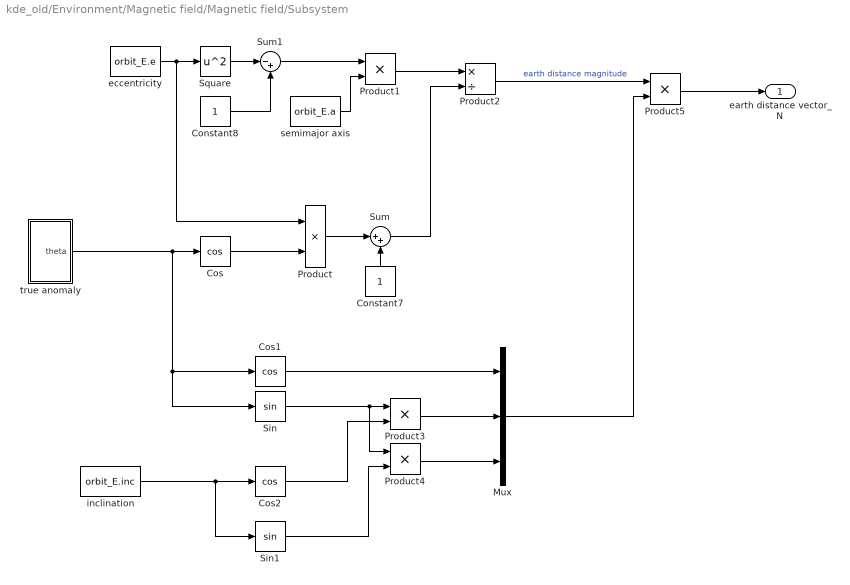
== system kde_old/Environment/Magnetic field/Magnetic field/Subsystem ==
  Constant7 : Constant
  Constant8 : Constant
  Cos : Trigonometry  Operator=cos
  Cos1 : Trigonometry  Operator=cos
  Cos2 : Trigonometry  Operator=cos
  Mux : Mux  Inputs=3
  Product{,1,3..5} (5 alike) : Product
  Product2 : Product  Inputs=*/
  Sin : Trigonometry
  Sin1 : Trigonometry
  Square : Math  Operator=square
  Sum : Sum  Inputs=|++
  Sum1 : Sum  Inputs=|-+
  eccentricity : Constant  Value=orbit_E.e
  inclination : Constant  Value=orbit_E.inc
  semimajor axis : Constant  Value=orbit_E.a
  true anomaly : Subsystem
  earth distance vector_N : Outport
  wires:
  Mux/1 -> Product5/2
  Product2/1 -> Product5/1  "earth distance magnitude"
  Product1/1 -> Product2/1
  Constant8/1 -> Sum1/2
  Sin/1 -> Product3/1, Product4/1
  true anomaly/1(theta) -> Sin/1, Cos1/1, Cos/1
  Cos/1 -> Product/2
  eccentricity/1 -> Product/1, Square/1
  Sin1/1 -> Product4/2
  Sum1/1 -> Product1/1
  Sum/1 -> Product2/2
  Product3/1 -> Mux/2
  Cos1/1 -> Mux/1
  Square/1 -> Sum1/1
  semimajor axis/1 -> Product1/2
  inclination/1 -> Sin1/1, Cos2/1
  Product4/1 -> Mux/3
  Constant7/1 -> Sum/2
  Product/1 -> Sum/1
  Product5/1 -> earth distance vector_N/1
  Cos2/1 -> Product3/2

== system kde_old/Environment/gravity gradient/Subsystem/true anomaly ==
  Constant : Constant  Value=orbit_E.theta0
  Constant1 : Constant  Value=orbit_E.n
  Constant10 : Constant  Value=3/2
  Constant8 : Constant
  Constant9 : Constant
  Cos : Trigonometry  Operator=cos
  Integrator : Integrator  InitialConditionSource=external
  Power : Math  Operator=pow
  Product1 : Product
  Product2 : Product
  Product3 : Product  Inputs=*/
  Square : Math  Operator=square
  Square1 : Math  Operator=square
  Sum : Sum  Inputs=|++
  Sum1 : Sum  Inputs=|-+
  eccentricity : Constant  Value=orbit_E.e
  theta : Outport
  wires:
  eccentricity/1 -> Square1/1, Product1/2
  Sum1/1 -> Power/1
  Product3/1 -> Integrator/1  "theta_dot"
  Constant9/1 -> Sum1/2
  Constant8/1 -> Sum/2
  Square1/1 -> Sum1/1
  Square/1 -> Product2/1
  Sum/1 -> Square/1
  Product2/1 -> Product3/1
  Cos/1 -> Product1/1
  Power/1 -> Product3/2
  Constant10/1 -> Power/2
  Integrator/1 -> theta/1, Cos/1  "theta"
  Constant/1 -> Integrator/2
  Product1/1 -> Sum/1
  Constant1/1 -> Product2/2

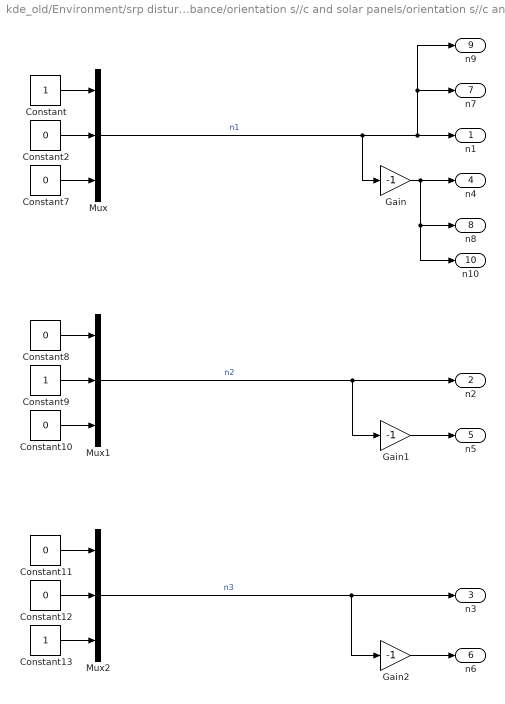
== system kde_old/Environment/srp disturbance/orientation s//c and solar panels/orientation s//c and solar panels in B ==
  Constant : Constant
  Constant{2,7..8,10..12} (6 alike) : Constant  Value=0
  Constant13 : Constant
  Constant9 : Constant
  Gain : Gain  Gain=-1
  Gain1 : Gain  Gain=-1
  Gain2 : Gain  Gain=-1
  Mux : Mux  Inputs=3
  Mux1 : Mux  Inputs=3
  Mux2 : Mux  Inputs=3
  n1 : Outport
  n2 : Outport  Port=2
  n3 : Outport  Port=3
  n4 : Outport  Port=4
  n5 : Outport  Port=5
  n6 : Outport  Port=6
  n7 : Outport  Port=7
  n8 : Outport  Port=8
  n9 : Outport  Port=9
  n10 : Outport  Port=10
  wires:
  Mux1/1 -> Gain1/1, n2/1  "n2"
  Mux2/1 -> n3/1, Gain2/1  "n3"
  Constant7/1 -> Mux/3
  Constant9/1 -> Mux1/2
  Gain1/1 -> n5/1
  Gain/1 -> n10/1, n8/1, n4/1
  Mux/1 -> Gain/1, n9/1, n7/1, n1/1  "n1"
  Constant11/1 -> Mux2/1
  Constant12/1 -> Mux2/2
  Gain2/1 -> n6/1
  Constant13/1 -> Mux2/3
  Constant10/1 -> Mux1/3
  Constant2/1 -> Mux/2
  Constant/1 -> Mux/1
  Constant8/1 -> Mux1/1

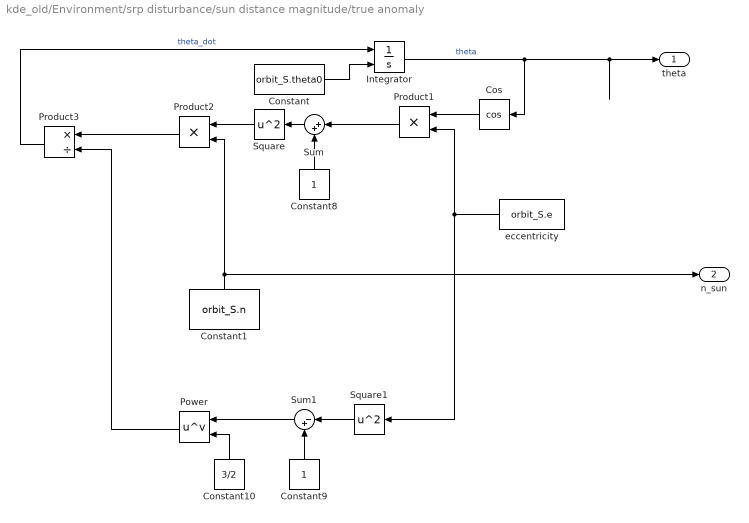
== system kde_old/Environment/srp disturbance/sun distance magnitude/true anomaly ==
  Constant : Constant  Value=orbit_S.theta0
  Constant1 : Constant  Value=orbit_S.n
  Constant10 : Constant  Value=3/2
  Constant8 : Constant
  Constant9 : Constant
  Cos : Trigonometry  Operator=cos
  Integrator : Integrator  InitialConditionSource=external
  Power : Math  Operator=pow
  Product1 : Product
  Product2 : Product
  Product3 : Product  Inputs=*/
  Square : Math  Operator=square
  Square1 : Math  Operator=square
  Sum : Sum  Inputs=|++
  Sum1 : Sum  Inputs=|-+
  eccentricity : Constant  Value=orbit_S.e
  theta : Outport
  n_sun : Outport  Port=2
  wires:
  Sum/1 -> Square/1
  Product1/1 -> Sum/1
  Integrator/1 -> theta/1, Cos/1  "theta"
  Cos/1 -> Product1/1
  Square/1 -> Product2/1
  Constant8/1 -> Sum/2
  Square1/1 -> Sum1/1
  eccentricity/1 -> Square1/1, Product1/2
  Constant10/1 -> Power/2
  Sum1/1 -> Power/1
  Constant9/1 -> Sum1/2
  Power/1 -> Product3/2
  Product3/1 -> Integrator/1  "theta_dot"
  Product2/1 -> Product3/1
  Constant/1 -> Integrator/2
  Constant1/1 -> n_sun/1, Product2/2

== system kde_old/Environment/Magnetic field/Magnetic field/Subsystem/true anomaly ==
  Constant : Constant  Value=orbit_E.theta0
  Constant1 : Constant  Value=orbit_E.n
  Constant10 : Constant  Value=3/2
  Constant8 : Constant
  Constant9 : Constant
  Cos : Trigonometry  Operator=cos
  Integrator : Integrator  InitialConditionSource=external
  Power : Math  Operator=pow
  Product1 : Product
  Product2 : Product
  Product3 : Product  Inputs=*/
  Square : Math  Operator=square
  Square1 : Math  Operator=square
  Sum : Sum  Inputs=|++
  Sum1 : Sum  Inputs=|-+
  eccentricity : Constant  Value=orbit_E.e
  theta : Outport
  wires:
  eccentricity/1 -> Square1/1, Product1/2
  Sum1/1 -> Power/1
  Product3/1 -> Integrator/1  "theta_dot"
  Constant9/1 -> Sum1/2
  Constant8/1 -> Sum/2
  Square1/1 -> Sum1/1
  Square/1 -> Product2/1
  Sum/1 -> Square/1
  Product2/1 -> Product3/1
  Cos/1 -> Product1/1
  Power/1 -> Product3/2
  Constant10/1 -> Power/2
  Integrator/1 -> theta/1, Cos/1  "theta"
  Constant/1 -> Integrator/2
  Product1/1 -> Sum/1
  Constant1/1 -> Product2/2

== matlab function kde_old/Attitude determination and control/Actuator/Subsystem1/MATLAB Function ==
  data: I input; u input; om input; om_dot output
function om_dot= fcn(I, u, om)

Ix = I(1); Iy = I(2); Iz = I(3);

om_dot_x = (Iy - Iz) / Ix * om(2) * om(1) + 1/Ix * u(1);
om_dot_y = (Iz - Ix) / Iy * om(1) * om(3) + 1/Iy * u(2); 
om_dot_z = (Ix - Iy) / Iz * om(1) * om(2) + 1/Iz * u(3);

om_dot = [om_dot_x, om_dot_y, om_dot_z]';

== matlab function kde_old/Attitude determination and control/Actuator/Subsystem1/MATLAB Function1 ==
  data: om input; dA output; A input
function dA = fcn(om, A)

om_hat = [  0,   -om(3),  om(2);
          om(3),   0,    -om(1); 
         -om(2),  om(1),   0];

dA = -om_hat * A;

== matlab function kde_old/Environment/srp disturbance/Subsystem/MATLAB Function1 ==
  data: F input; pos input; T_SRP output; cond input
function T_SRP = fcn(F, pos, cond)

T = zeros(length(cond),3);

for i = 1:length(cond)
    if cond(i) > 0
        T(i,:) = cross(pos(:,i), F(:,i));
    end
end

T_sum = sum(T);

T_SRP = T_sum;

== matlab function kde_old/Attitude determination and control/Actuator/Subsystem1/MATLAB Function2 ==
  data: om input; u output; Ae input; k1 input; k2 input
function u = fcn(om, Ae, k1, k2)

Ae_diff = Ae' - Ae;

alpha = [Ae_diff(3, 1), Ae_diff(1, 3), Ae_diff(2, 1)]';

u1 = - k1 * om(1) - k2 * alpha(1);
u2 = - k1 * om(2) - k2 * alpha(2);
u3 = - k1 * om(3) - k2 * alpha(3);

u = [u1, u2, u3]';
